simulink model "control_system_smc"  (R2025b)
settings: Solver=VariableStepAuto  StartTime=0.0  StopTime=20  FixedStep=0.01  MaxStep=0.001  RelTol=1e-3
values from neighbouring files (symbols this model uses):
  A1 = 0    [init_control_system_smc.m]
  A2 = 0    [init_control_system_smc.m]
  k = 15    [init_control_system_smc.m]
  k_law = 1    [init_control_system_smc.m]
  p1 = 1    [init_control_system_smc.m]
  p2 = -1    [init_control_system_smc.m]
  x0 = [1 1.5]'    [init_control_system_smc.m]
  x1d = 2.7081    [init_control_system_smc.m]
  x2d = 2.7081    [init_control_system_smc.m]
libraries: simulink x1
settings Model: Creator=ricca  LastModifiedBy=ricca

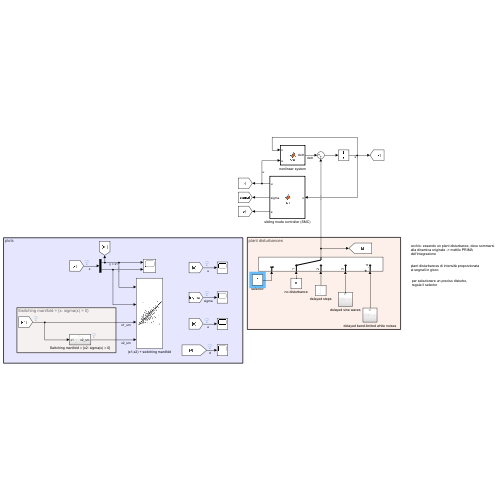
[thumbnail: Simulink's stored preview of the top-level diagram]
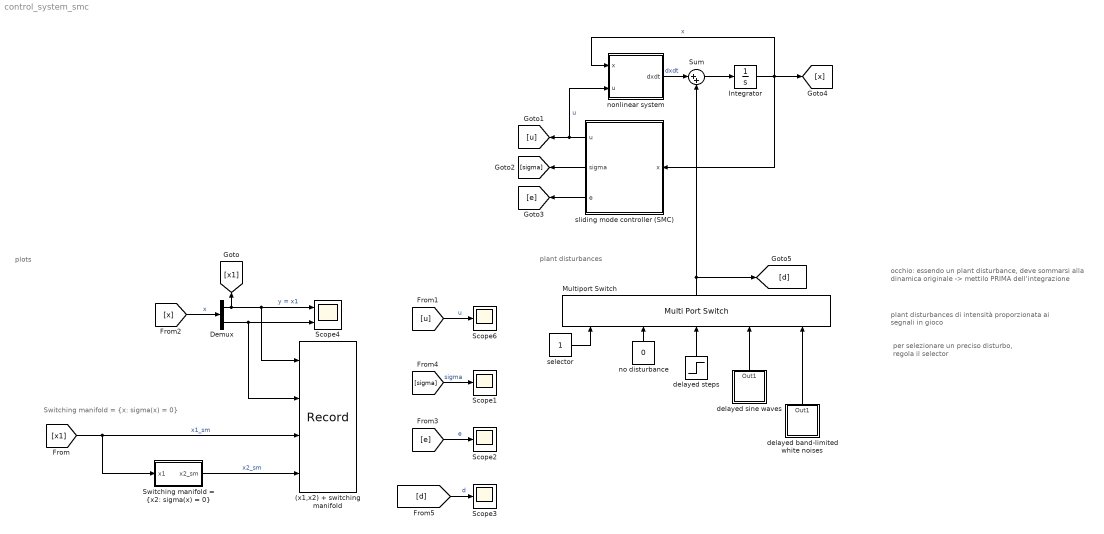
== system control_system_smc ==
  note: Switching manifold = {x: sigma(x) = 0}
  note: plots
  note: plant disturbances
  note: occhio: essendo un plant disturbance, deve sommarsi alla dinamica originale -> mettilo PRIMA dell'integrazione
  note: per selezionare un preciso disturbo, regola il selector
  note: plant disturbances di intensità proporzionata ai segnali in gioco
  (x1,x2) + switching manifold : Record  NumPorts=4.0  FileSettingsInternal="{\"entries\":[{\"content\":{\"excelSettings\":{\"content\":{},\"type\":\"Streamout.ExcelSettings\"},\"parquetSettings\":{\"content\":{},\"type\":\"Streamout.ParquetSettings\"}},\"type\":\"Streamout.FileSettingStorage\",\"uuid\":\"\"}],\"packageUris\":[\"http:\\/\\/schema.mathworks.com\\/mf0\\/streamout_blocks\\/R2020a\"],\"version\":\"1.0\"}"  FrameSettings=[0, 0, 0, 0]  Layout=[1 1]  SignalsInternal="{\"entries\":[{\"content\":{\"signals\":[{\"content\":{\"blockPath\":[],\"dimensions\":[1],\"domain\":\"\",\"lineColor\":\"#139fff\",\"plots\":[ 1 ],\"port\":1,\"sid\":[\"\"],\"signalID\":1,\"signalName\":\"y = x1\"},\"type\":\"RecordBlkView.Signal\",\"uuid\":\"\"},{\"content\":{\"blockPath\":[],\"dimensions\":[1],\"domain\":\"\",\"lineColor\":\"#139fff\",\"plots\":[ 1 ],\"port\":2,\"sid\":[\"\"],\"signalID\":2,\"signalName\":\"Demux:2\"},\"type\":\"RecordBlkView.Signal\",\"uuid\":\"\"},{\"content\":{\"blockPath\":[],\"dimensions\":[1],\"domain\":\"\",\"lineColor\":\"#a2142f\",\"lineWidth\":20,\"plots\":[ 1 ],\"port\":3,\"sid\":[\"\"],\"signalID\":3,\"signalName\":\"x1_sm\"},\"type\":\"RecordBlkView.Signal\",\"uuid\":\"\"},{\"content\":{\"blockPath\":[],\"dimensions\":[1],\"domain\":\"\",\"lineColor\":\"#a2142f\",\"lineWidth\":20,\"plots\":[ 1 ],\"port\":4,\"sid\":[\"\"],\"signalID\":4,\"signalName\":\"x2_sm\"},\"type\":\"RecordBlkView.Signal\",\"uuid\":\"\"}]},\"type\":\"RecordBlkView.InputSignals\",\"uuid\":\"\"}],\"packageUris\":[\"http:\\/\\/schema.mathworks.com\\/mf0\\/streamout_blocks\\/R2020a\"],\"version\":\"1.0\"}"  VisualizationBindings="{\"xyplotplugin\":{\"info\":[{\"series\":[{\"bindingParametersList\":[{\"parameter\":\"X-Axis\",\"signalID\":3,\"signalName\":\"x1_sm\"},{\"parameter\":\"Y-Axis\",\"signalID\":4,\"signalName\":\"x2_sm\"}],\"seriesID\":0},{\"bindingParametersList\":[{\"parameter\":\"X-Axis\",\"signalID\":1,\"signalName\":\"y = x1\"},{\"parameter\":\"Y-Axis\",\"signalID\":2,\"signalName\":\"Demux:2\"}],\"seriesID\":1}],\"subplotID\":1}]}}"  CompatibilityTag=XY
  Demux : Demux  Outputs=2
  Integrator : Integrator  InitialCondition=x0
  Multiport Switch : MultiPortSwitch  Inputs=4  SaturateOnIntegerOverflow=off  InputSameDT=off
  Scope{1..3,6} (4 alike) : Scope
      Scope1 settings: ActiveDisplayYMinimum=-0.53894481328193644  ActiveDisplayYMaximum=0.059753173159124089
      Scope2 settings: ActiveDisplayYMinimum=-0.53894481328193644  ActiveDisplayYMaximum=0.059753173159124089
      Scope3 settings: ActiveDisplayYMinimum=-0.074999999999999983  ActiveDisplayYMaximum=0.67499999999999993  DataLoggingVariableName=ScopeData2
      Scope6 settings: ActiveDisplayYMinimum=-1.559270928041987  ActiveDisplayYMaximum=1.2852401244230949  DataLoggingVariableName=ScopeData3
  Scope4 : Scope  NumInputPorts=2
      settings: ActiveDisplayYMinimum=0.76201934452175279  ActiveDisplayYMaximum=3.1418258993042252  DataLoggingVariableName=ScopeData4
  Sum : Sum  Inputs=|++
  "Switching manifold = {x2: sigma(x) = 0}" : Subsystem
  delayed band-limited white noises : Subsystem
  delayed sine waves : Subsystem
  delayed steps : Step  Time=[7 8]'  After=[0.5 0.6]'  SampleTime=0
  no disturbance : Constant  Value=0  OutDataTypeStr=Inherit: Inherit via back propagation
  nonlinear system : MATLAB Function  TreatAsAtomicUnit=on
  selector : Constant
  sliding mode controller (SMC) : MATLAB Function  TreatAsAtomicUnit=on
  wires:
  Integrator/1 -> sliding mode controller (SMC)/1(x), [x], nonlinear system/1(x)  "x"
  [x1] -> (x1,x2) + switching manifold/3, "Switching manifold = {x2: sigma(x) = 0}"/1(x1)  "x1_sm"
  sliding mode controller (SMC)/1(u) -> [u], nonlinear system/2(u)  "u"
  "Switching manifold = {x2: sigma(x) = 0}"/1(x2_sm) -> (x1,x2) + switching manifold/4  "x2_sm"
  Demux/2 -> (x1,x2) + switching manifold/2, Scope4/2
  Demux/1 -> (x1,x2) + switching manifold/1, Scope4/1, [x1]  "y = x1"
  [u] -> Scope6/1  "u"
  [sigma] -> Scope1/1  "sigma"
  nonlinear system/1(dxdt) -> Sum/1  "dxdt"
  [x] -> Demux/1  "x"
  [e] -> Scope2/1  "e"
  sliding mode controller (SMC)/2(sigma) -> [sigma]
  sliding mode controller (SMC)/3(e) -> [e]
  Sum/1 -> Integrator/1
  [d] -> Scope3/1  "d"
  selector/1 -> Multiport Switch/1
  delayed sine waves/1(Out1) -> Multiport Switch/4
  Multiport Switch/1 -> Sum/2, [d]
  no disturbance/1 -> Multiport Switch/2
  delayed band-limited white noises/1(Out1) -> Multiport Switch/5
  delayed steps/1 -> Multiport Switch/3

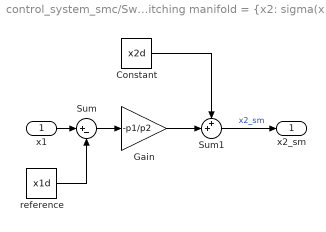
== system control_system_smc/Switching manifold = {x2: sigma(x) = 0} ==
  x1 : Inport
  Constant : Constant  Value=x2d
  Gain : Gain  Gain=-p1/p2
  Sum : Sum  Inputs=|+-
  Sum1 : Sum  Inputs=++|
  reference : Constant  Value=x1d
  x2_sm : Outport
  wires:
  Sum1/1 -> x2_sm/1  "x2_sm"
  Sum/1 -> Gain/1
  x1/1 -> Sum/1
  reference/1 -> Sum/2
  Gain/1 -> Sum1/2
  Constant/1 -> Sum1/1

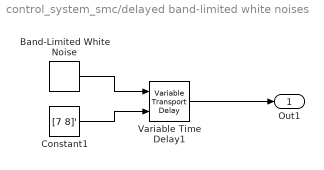
== system control_system_smc/delayed band-limited white noises ==
  Band-Limited White Noise : simulink/Sources/Band-Limited White Noise  Cov=[0.01 0.01]'  Ts=0.1  seed=[23341 23342]'
  Constant1 : Constant  Value=[7 8]'
  Variable Time Delay1 : VariableTransportDelay  MaximumDelay=10
  Out1 : Outport
  wires:
  Constant1/1 -> Variable Time Delay1/2
  Band-Limited White Noise/1 -> Variable Time Delay1/1
  Variable Time Delay1/1 -> Out1/1

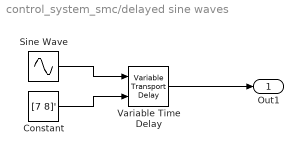
== system control_system_smc/delayed sine waves ==
  Constant : Constant  Value=[7 8]'
  Sine Wave : Sin  Amplitude=[0.5 0.6]'  Bias=[0 0]'  SampleTime=0
  Variable Time Delay : VariableTransportDelay  MaximumDelay=10
  Out1 : Outport
  wires:
  Sine Wave/1 -> Variable Time Delay/1
  Variable Time Delay/1 -> Out1/1
  Constant/1 -> Variable Time Delay/2

== matlab function control_system_smc/nonlinear system ==
  data: x input; u input; dxdt output size=2; A1 parameter; A2 parameter; k parameter
function dxdt = fcn(x,u,A1,A2,k)

dxdt = [-x(1) + A2 + k*x(2)*exp(-x(2));           
        -x(2) + A1 + k*x(1)*exp(-x(1)) + u];    

%% se vuoi testare le capacità di robustezza rispetto a unmodelled dynamics  Delta_f, uncommmenta i Delta_f e dxdt sotto, e commmenta il dxdt sopra. Ricordati di aumentare k_law, come da teoria!

% Delta_f = 0.2*sin(x(1));
% dxdt = [-x(1) + A2 + k*x(2)*exp(-x(2)) + Delta_f;           
%         -x(2) + A1 + k*x(1)*exp(-x(1)) + Delta_f + u];    

%% se vuoi testare le capacità di robustezza rispetto a parametric uncertainties del 10% su k, uncommmenta dxdt sotto, e commmenta il dxdt sopra.

% dxdt = [-x(1) + A2 + (k+0.10*k)*x(2)*exp(-x(2));           
%         -x(2) + A1 + (k+0.10*k)*x(1)*exp(-x(1)) + u];    


end

== matlab function control_system_smc/sliding mode controller (SMC) ==
  data: x input; u output; p1 parameter; p2 parameter; k_law parameter; x1d parameter; x2d parameter; A1 parameter; A2 parameter; k parameter; sigma output; e output
function [u,sigma,e] = fcn(x,p1,p2, k_law, x1d,x2d, A1, A2, k)

% sigma, Lgsigma e Lfsigma copiati e incollati dai risultati di "init_control_system_smc.m"
sigma = p1*(x(1) - x1d) + p2*(x(2) - x2d);
Lgsigma = p2;
Lfsigma = p2*(A1 - x(2) + k*x(1)*exp(-x(1))) + p1*(A2 - x(1) + k*x(2)*exp(-x(2)));

u = 1/Lgsigma*(-Lfsigma - k_law*sign(sigma));      % ideal version of the control law 
%u = 1/Lgsigma*(-Lfsigma - k_law*sat(sigma/0.03)); % chattering-reducing version of the control law. 

e = x1d - x(1);

end


% saturation function
function y=sat(x)
    if abs(x) <= 1
        y = x;
    else
        y = sign(x);
    end
end


% Gli effetti dell'utilizzo di sat() è problem dependent!
% The slope of the linear portion of sat(x/eps) is 1/eps. Good 
% approximation requires the use of small eps. In the limit, as eps -> 0, 
% the saturation function sat(x/eps) approaches the signum function sgn(x).
% For better accuracy, we need to choose eps as small as possible, but a 
% too small value of eps will induce chattering in the presence of time 
% delays or unmodeled fast dynamics.
